simulink library "target_generation_lib"  (R2016b)
settings: Solver=VariableStepAuto  StartTime=0.0  StopTime=10.0  RelTol=1e-3
settings Model: Creator=taylorreynolds  LastModifiedBy=bijan

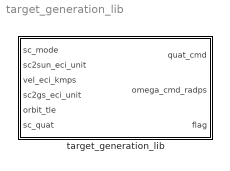
== system target_generation_lib ==
  target_generation_lib : Subsystem

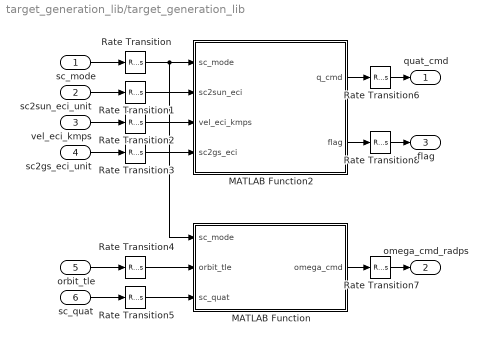
== system target_generation_lib/target_generation_lib ==
  sc_mode : Inport
  sc2sun_eci_unit : Inport  Port=2
  vel_eci_kmps : Inport  Port=3
  sc2gs_eci_unit : Inport  Port=4
  orbit_tle : Inport  Port=5
  sc_quat : Inport  Port=6
  MATLAB Function : MATLAB Function  TreatAsAtomicUnit=on
  MATLAB Function2 : MATLAB Function  TreatAsAtomicUnit=on
  Rate Transition : RateTransition  X0=fsw_params.target_gen.ic.sc_mode  OutPortSampleTime=fsw_params.target_gen.sample_time_s
  Rate Transition{1..5} (5 alike) : RateTransition  OutPortSampleTime=fsw_params.target_gen.sample_time_s
  Rate Transition6 : RateTransition  X0=fsw_params.target_gen.ic.quat
  Rate Transition7 : RateTransition  X0=fsw_params.target_gen.ic.omega
  Rate Transition8 : RateTransition  X0=fsw_params.target_gen.ic.flag
  quat_cmd : Outport
  omega_cmd_radps : Outport  Port=2
  flag : Outport  Port=3
  wires:
  MATLAB Function2/1(q_cmd) -> Rate Transition6/1
  sc2gs_eci_unit/1 -> Rate Transition3/1
  vel_eci_kmps/1 -> Rate Transition2/1
  sc2sun_eci_unit/1 -> Rate Transition1/1
  orbit_tle/1 -> Rate Transition4/1
  sc_quat/1 -> Rate Transition5/1
  MATLAB Function/1(omega_cmd) -> Rate Transition7/1
  sc_mode/1 -> Rate Transition/1
  Rate Transition/1 -> MATLAB Function/1(sc_mode), MATLAB Function2/1(sc_mode)
  Rate Transition1/1 -> MATLAB Function2/2(sc2sun_eci)
  Rate Transition2/1 -> MATLAB Function2/3(vel_eci_kmps)
  Rate Transition3/1 -> MATLAB Function2/4(sc2gs_eci)
  Rate Transition4/1 -> MATLAB Function/2(orbit_tle)
  Rate Transition5/1 -> MATLAB Function/3(sc_quat)
  Rate Transition6/1 -> quat_cmd/1
  Rate Transition7/1 -> omega_cmd_radps/1
  MATLAB Function2/2(flag) -> Rate Transition8/1
  Rate Transition8/1 -> flag/1

== matlab function target_generation_lib/MATLAB Function ==
  data: sc_mode input size=1; omega_cmd output size=3; orbit_tle input size=9; sc_quat input size=4
 function omega_cmd = fcn(sc_mode,orbit_tle,sc_quat)
%#codegen
% FSW Target Generation Library
%   UW HuskySat-1, ADCS Team
%   Last Updated: T. Reynolds 1.15.18

% Computes desired quaternion and angular velocity depending on the sc_mode
%   mode_logic.bdot             = 1;
%   mode_logic.desat_eclipse    = 2;
%   mode_logic.point            = 3;
%       point.velocity          = 31;
%       point.ground            = 32;
%       point.MPC               = 33;
%   mode_logic.low_power        = 4;

XSPDA   = 86400;        % seconds per day
DE2RA   = 0.174532925e-1;   % radians/degree

n_orb   = [0;0;orbit_tle(9)*2*pi/XSPDA]; % mean motion [rad/s]
INC     = orbit_tle(4)*DE2RA; % inclination [rad]
RAAN    = orbit_tle(5)*DE2RA; % right ascension of ascending node [rad]
AOP     = orbit_tle(7)*DE2RA; % argument of perigee [rad]

C_orb2eci   = rot3(-RAAN)*rot1(-INC)*rot3(-AOP);
n_eci   = C_orb2eci*n_orb;

C_eci2body  = quat2DCM(sc_quat);
n_body  = C_eci2body'*n_eci;

if( sc_mode == 31 || sc_mode == 32 )
    % Commanded Angular Velocity
    omega_cmd   = n_body;
else
    % Commanded Angular Velocity
    omega_cmd   = zeros(3,1);
end


end

function C1 = rot1( ang )
    C1  = [ ...
            1   0           0;
            0   cos(ang)    sin(ang);
            0   -sin(ang)   cos(ang) ];
end

% function C2 = rot2( ang )
%     C2  = [ ...
%             cos(ang)    0   -sin(ang);
%             0           1   0;
%             sin(ang)    0   cos(ang) ];
% end

function C3 = rot3( ang )
    C3  = [ ...
            cos(ang)    sin(ang)    0;
            -sin(ang)   cos(ang)    0;
            0           0           1 ];
end

function DCM = quat2DCM( q )
    q0  = q(1);
    qv  = reshape(q(2:4),3,1);
    
    DCM     = (2*q0^2 - 1)*eye(3) + 2*(qv*qv') - 2*q0*skew(qv);
    
end

== matlab function target_generation_lib/MATLAB Function2 ==
  data: sc_mode input size=1; q_cmd output size=4; sc2sun_eci input size=3; vel_eci_kmps input size=3; sc2gs_eci input size=3; flag output
  function [q_cmd,flag]   = TRIAD(sc_mode,sc2sun_eci,vel_eci_kmps,sc2gs_eci)
%#codegen
% FSW Target Generation Library
%   UW HuskySat-1, ADCS Team
%   Last Updated: T. Reynolds 1.15.18

% Computes desired quaternion and angular velocity depending on the sc_mode
%   mode_logic.bdot             = 1;
%   mode_logic.desat_eclipse    = 2;
%   mode_logic.point            = 3;
%       point.velocity          = 31;
%       point.ground            = 32;
%       point.MPC               = 33;
%   mode_logic.low_power        = 4;

COM2    = [0; -1; 0];
PPT     = [0; 0; -1];
flag = 0;
tol = 1e-3;

% PPT     = [0;1;2];    % these are used for testing only
% SP      = [1;3;0];

Cx5  = [ 1 0 0; 0 cosd(5) sind(5); 0 -sind(5) cosd(5)];

% Check for zero vectors
if( norm(vel_eci_kmps) < tol || norm(sc2sun_eci) < tol || norm(sc2gs_eci) < tol )
    flag = -1;
end

if( sc_mode == 31 && flag == 0 )
    
    SP  = [0; 1; 0];
    
    % Body
    B1  = PPT./norm(PPT);
    B2  = SP./norm(SP);
    Xtb     = B1;
    Ytb     = cross(B1,B2)/norm(cross(B1,B2));
    Ztb     = cross(B1,cross(B1,B2))/norm(cross(B1,B2));
    
    % Inertial
    S1  = vel_eci_kmps./norm(vel_eci_kmps);
    S2  = sc2sun_eci./norm(sc2sun_eci);
    Xti     = S1;
    Yti     = cross(S1,S2)/norm(cross(S1,S2));
    Zti     = cross(S1,cross(S1,S2))/norm(cross(S1,S2));
    
    % Stack vectors
    Cb  = [Xtb, Ytb, Ztb];
    Ci  = [Xti, Yti, Zti];
    
    % Commanded DCM ( body to inertial )
    C_cmd   = Ci*Cb';
        
elseif( sc_mode == 32 && flag == 0 )
    
    % Tilted so doesn't aling with COM2 -- chose a 5[deg] roll.
    SP      = Cx5*[0;1;0]; 
    
    % Body
    B1  = COM2./norm(COM2);
    B2  = SP./norm(SP);
    Xtb     = B1;
    Ytb     = cross(B1,B2)/norm(cross(B1,B2));
    Ztb     = cross(B1,cross(B1,B2))/norm(cross(B1,B2));
    
    % Inertial
    S1  = sc2gs_eci./norm(sc2gs_eci);
    S2  = sc2sun_eci./norm(sc2sun_eci);
    Xti     = S1;
    Yti     = cross(S1,S2)/norm(cross(S1,S2));
    Zti     = cross(S1,cross(S1,S2))/norm(cross(S1,S2));
    
    % Stack vectors
    Cb  = [Xtb, Ytb, Ztb];
    Ci  = [Xti, Yti, Zti];
    
    % Commanded DCM ( body to inertial )
    C_cmd   = Ci*Cb';
    
else
    C_cmd   = eye(3);
end

% Compute commanded quaternion from DCM
q_cmd   = myDCM2quat( C_cmd );

end


% function q = DCM2quat( dcm )
%     q   = zeros(4,1);
%     
%     tr = trace(dcm);
% 
%     if (tr > 0)
%         sqtrp1 = sqrt( tr + 1.0 );
%         
%         q(1) = 0.5*sqtrp1; 
%         q(2) = (dcm(2, 3) - dcm(3, 2))/(2.0*sqtrp1);
%         q(3) = (dcm(3, 1) - dcm(1, 3))/(2.0*sqtrp1); 
%         q(4) = (dcm(1, 2) - dcm(2, 1))/(2.0*sqtrp1); 
%     else
%         d = diag(dcm);
%         if ((d(2) > d(1)) && (d(2) > d(3)))
%             % max value at dcm(2,2)
%             sqdip1 = sqrt(d(2) - d(1) - d(3) + 1.0 );
%             
%             q(3) = 0.5*sqdip1; 
%             
%             if ( sqdip1 ~= 0 )
%                 sqdip1 = 0.5/sqdip1;
%             end
%             
%             q(1) = (dcm(3, 1) - dcm(1, 3))*sqdip1; 
%             q(2) = (dcm(1, 2) + dcm(2, 1))*sqdip1; 
%             q(4) = (dcm(2, 3) + dcm(3, 2))*sqdip1; 
%         elseif (d(3) > d(1))
%             % max value at dcm(3,3)
%             sqdip1 = sqrt(d(3) - d(1) - d(2) + 1.0 );
%             
%             q(4) = 0.5*sqdip1; 
%             
%             if ( sqdip1 ~= 0 )
%                 sqdip1 = 0.5/sqdip1;
%             end
%             
%             q(1) = (dcm(1, 2) - dcm(2, 1))*sqdip1;
%             q(2) = (dcm(3, 1) + dcm(1, 3))*sqdip1; 
%             q(3) = (dcm(2, 3) + dcm(3, 2))*sqdip1; 
%         else
%             % max value at dcm(1,1)
%             sqdip1 = sqrt(d(1) - d(2) - d(3) + 1.0 );
%             
%             q(2) = 0.5*sqdip1; 
%             
%             if ( sqdip1 ~= 0 )
%                 sqdip1 = 0.5/sqdip1;
%             end
%             
%             q(1) = (dcm(2, 3) - dcm(3, 2))*sqdip1; 
%             q(3) = (dcm(1, 2) + dcm(2, 1))*sqdip1; 
%             q(4) = (dcm(3, 1) + dcm(1, 3))*sqdip1; 
%         end
% 
%     end
% 
% end

function q = myDCM2quat( DCM )

q   = zeros(4,1);

tr  = trace(DCM);

q(1)    = 0.5*sqrt(tr + 1);

if( q(1) ~= 0 )
    eta     = 1/(4*q(1));
    q(2)    = eta*(DCM(2,3) - DCM(3,2));
    q(3)    = eta*(DCM(3,1) - DCM(1,3));
    q(4)    = eta*(DCM(1,2) - DCM(2,1));
else
    q(2)  = sqrt(0.5*(DCM(1,1) + 1));
    q(3)  = sign(DCM(1,2))*sqrt(0.5*(DCM(2,2) + 1));
    q(4)  = sign(DCM(1,3))*sqrt(0.5*(DCM(3,3) + 1));
end


end
